simulink model "table_test"  (R2025a)
settings: Solver=ode4  StartTime=0.0  StopTime=Stop_Time  FixedStep=1e-5  RelTol=1e-3
values from neighbouring files (symbols this model uses):
  B = 2/n*trapz(y.*sin(o*theta))    [ch04_half_inverter.m]
  Lamf = 0.32    [SPMSM_MTPA_plot.m]    (also in a_OpenLoop_IPMSM.m = 0.12; a_OpenLoop_SPMSM.m = 0.31; ch03_SPMSM_MTPA_plot.m = 0.28; ch03_control_MTPA_plot.m = 0.12)
  Lds = 30e-3    (= 0.03)    [SPMSM_MTPA_plot.m]    (also in a_OpenLoop_IPMSM.m; a_OpenLoop_SPMSM.m; ch03_SPMSM_MTPA_plot.m; ch03_contour_colorful.m = 0.000243)
  Lqs = 30e-3    (= 0.03)    [SPMSM_MTPA_plot.m]    (also in a_OpenLoop_IPMSM.m = 0.04; a_OpenLoop_SPMSM.m; ch03_SPMSM_MTPA_plot.m; ch03_contour_colorful.m = 0.000298)
  P = 24    [SPMSM_MTPA_plot.m]    (also in a_OpenLoop_IPMSM.m; a_OpenLoop_SPMSM.m; ch03_SPMSM_MTPA_plot.m; ch03_contour_colorful.m = 8)
  Rs = 0.22    [chapter04_ff.m]
undefined symbols (not defined in the file or in its folder): J, Kic, Kpc
settings Model: Creator=New  LastModifiedBy=New

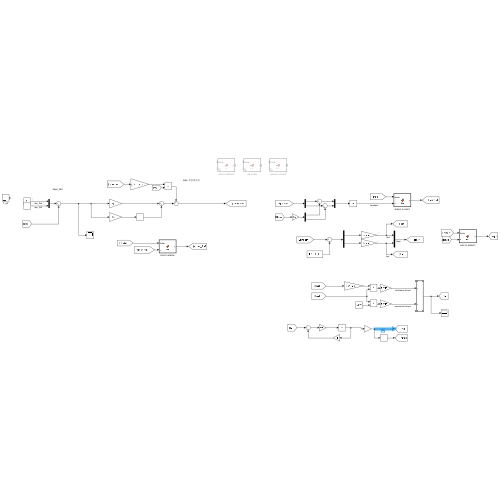
[thumbnail: Simulink's stored preview of the top-level diagram]
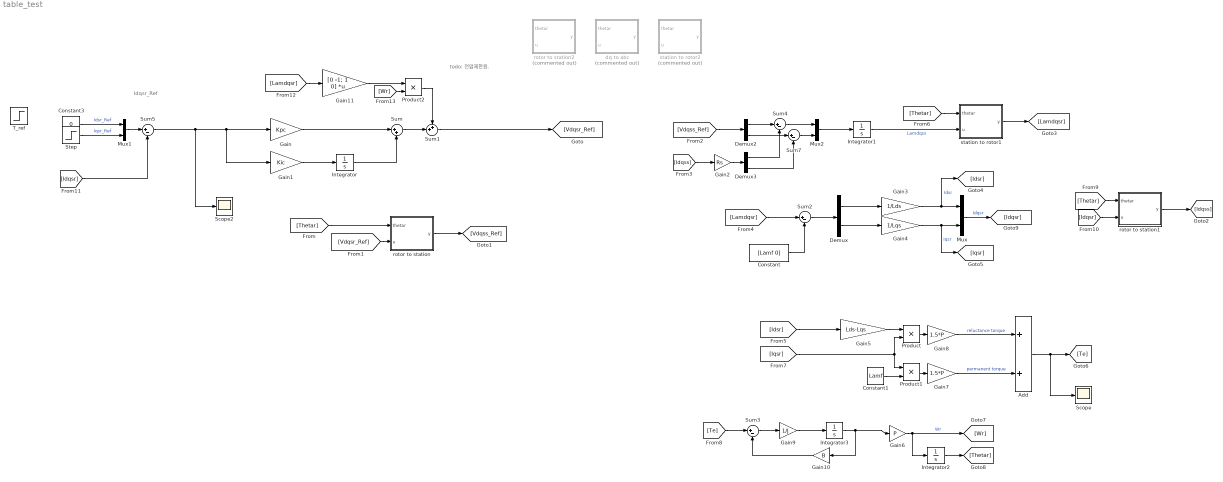
== system table_test ==
  note: Idqsr_Ref
  note: todo: 전압제한원.
  Add : Sum
  Constant : Constant  Value=[Lamf 0]
  Constant1 : Constant  Value=Lamf
  Constant3 : Constant  Value=0
  Demux : Demux  Outputs=2
  Demux2 : Demux  Outputs=2
  Demux3 : Demux  Outputs=2
  Gain : Gain  Gain=Kpc
  Gain1 : Gain  Gain=Kic
  Gain10 : Gain  Gain=B
  Gain11 : Gain  Gain=[0 -1; 1 0]  Multiplication=Matrix(K*u)
  Gain2 : Gain  Gain=Rs
  Gain3 : Gain  Gain=1/Lds
  Gain4 : Gain  Gain=1/Lqs
  Gain5 : Gain  Gain=Lds-Lqs
  Gain6 : Gain  Gain=P
  Gain7 : Gain  Gain=1.5*P
  Gain8 : Gain  Gain=1.5*P
  Gain9 : Gain  Gain=1/J
  Integrator{,1..3} (4 alike) : Integrator
  Mux : Mux  Inputs=2
  Mux1 : Mux  Inputs=2
  Mux2 : Mux  Inputs=2
  Product : Product
  Product1 : Product
  Product2 : Product
  Scope : Scope
      settings: ActiveDisplayYMinimum=-1.9971388409869073  ActiveDisplayYMaximum=17.974249568882168
  Scope2 : Scope
      settings: ActiveDisplayYMinimum=-1.3031281364153293  ActiveDisplayYMaximum=4.589236459601703  DataLoggingVariableName=ScopeData2
  Step : Step  Time=0.1  After=4  SampleTime=0
  Sum : Sum  Inputs=|++
  Sum1 : Sum  Inputs=++|
  Sum{2..5,7} (5 alike) : Sum  Inputs=|+-
  T_ref : Step  SampleTime=0
  dq to abc : MATLAB Function  Commented=on  TreatAsAtomicUnit=on
  rotor to station : MATLAB Function  TreatAsAtomicUnit=on
  rotor to station1 : MATLAB Function  TreatAsAtomicUnit=on
  rotor to station2 : MATLAB Function  Commented=on  TreatAsAtomicUnit=on
  station to rotor1 : MATLAB Function  TreatAsAtomicUnit=on
  station to rotor2 : MATLAB Function  Commented=on  TreatAsAtomicUnit=on
  wires:
  Gain1/1 -> Integrator/1
  Gain/1 -> Sum/1
  Integrator/1 -> Sum/2
  [Thetar] -> rotor to station/1(thetar)
  [Vdqsr_Ref] -> rotor to station/2(u)
  rotor to station/1(y) -> [Vdqss_Ref]
  [Idqss] -> Gain2/1
  Mux2/1 -> Integrator1/1
  Integrator1/1 -> station to rotor1/2(u)  "Lamdqss"
  [Thetar] -> station to rotor1/1(thetar)
  station to rotor1/1(y) -> [Lamdqsr]
  [Lamdqsr] -> Sum2/1
  Constant/1 -> Sum2/2
  Sum2/1 -> Demux/1
  Demux/1 -> Gain3/1
  Demux/2 -> Gain4/1
  Gain3/1 -> Mux/1, [Idsr]  "Idsr"
  Gain4/1 -> Mux/2, [Iqsr]  "Iqsr"
  [Idsr] -> Gain5/1
  Gain5/1 -> Product/1
  [Iqsr] -> Product/2, Product1/1
  Constant1/1 -> Product1/2
  Product/1 -> Gain8/1
  Product1/1 -> Gain7/1
  Add/1 -> Scope/1, [Te]
  Gain7/1 -> Add/2  "permanent torque"
  Gain8/1 -> Add/1  "reluctance torque"
  Integrator3/1 -> Gain10/1, Gain6/1
  Gain6/1 -> Integrator2/1, [Wr]  "Wr"
  Integrator2/1 -> [Thetar]
  [Thetar] -> rotor to station1/1(thetar)
  rotor to station1/1(y) -> [Idqss]
  Gain9/1 -> Integrator3/1
  Sum3/1 -> Gain9/1
  [Te] -> Sum3/1
  Gain10/1 -> Sum3/2
  [Idqsr] -> rotor to station1/2(u)
  Mux/1 -> [Idqsr]  "Idqsr"
  [Idqsr] -> Sum5/2
  [Vdqss_Ref] -> Demux2/1
  Gain2/1 -> Demux3/1
  Demux2/1 -> Sum4/1
  Demux3/1 -> Sum4/2
  Demux2/2 -> Sum7/1
  Demux3/2 -> Sum7/2
  Sum7/1 -> Mux2/2
  Sum4/1 -> Mux2/1
  Constant3/1 -> Mux1/1  "Idsr_Ref"
  Step/1 -> Mux1/2  "Iqsr_Ref"
  Mux1/1 -> Sum5/1
  Sum5/1 -> Scope2/1, Gain1/1, Gain/1
  Sum/1 -> Sum1/2
  Sum1/1 -> [Vdqsr_Ref]
  [Lamdqsr] -> Gain11/1
  Gain11/1 -> Product2/1
  [Wr] -> Product2/2
  Product2/1 -> Sum1/1

== matlab function table_test/rotor to station ==
  data: thetar input; y output; u input
function y = fcn(thetar, u)

T = [cos(thetar) -sin(thetar); 
     sin(thetar)  cos(thetar)];

y = T*u;

== matlab function table_test/rotor to station1 ==
  data: thetar input; y output; u input
function y = fcn(thetar, u)

T = [cos(thetar) -sin(thetar); 
     sin(thetar)  cos(thetar)];

y = T*u;

== matlab function table_test/station to rotor1 ==
  data: thetar input; y output; u input
function y = fcn(thetar, u)

T = [cos(thetar)  sin(thetar); 
    -sin(thetar)  cos(thetar)];

y = T*u;

== matlab function table_test/rotor to station2 ==
  data: thetar input; y output; u input
function y = fcn(thetar, u)

T = [cos(thetar) -sin(thetar); 
     sin(thetar)  cos(thetar)];

y = T*u;

== matlab function table_test/station to rotor2 ==
  data: thetar input; y output; u input
function y = fcn(thetar, u)

T = [cos(thetar)  sin(thetar); 
    -sin(thetar)  cos(thetar)];

y = T*u;

== matlab function table_test/dq to abc ==
  data: thetar input; y output; u input
function y = fcn(thetar, u)

a = 2*pi/3;
T =[cos(thetar)  cos(thetar-a)  cos(thetar+a);
   -sin(thetar) -sin(thetar-a) -sin(thetar+a);] *2/3;

y = T \ u;
